simulink model "Lab1_Exercise2_BD"  (R2023b)
settings: Solver=VariableStepAuto  StartTime=0.0  StopTime=100  RelTol=1e-3
settings Model: Creator=julia  LastModifiedBy=julia

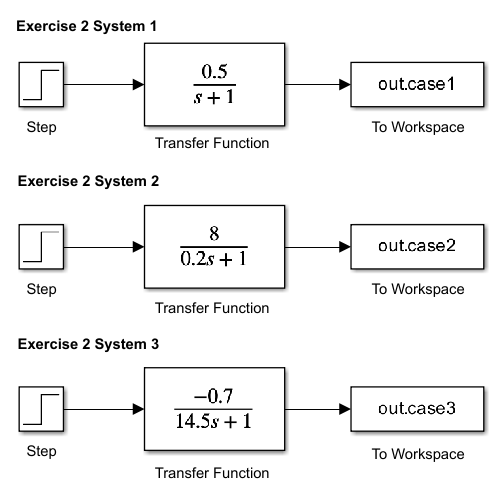
[thumbnail: Simulink's stored preview of the top-level diagram]
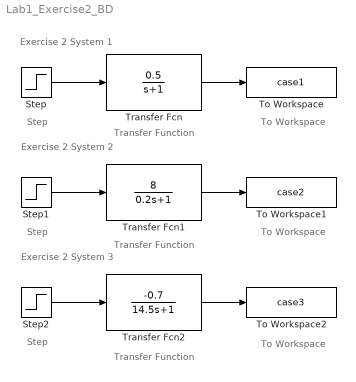
== system Lab1_Exercise2_BD ==
  note: Exercise 2 System 1
  note: Transfer Function
  note: To Workspace
  note: Step
  note: Step
  note: Step
  note: To Workspace
  note: To Workspace
  note: Transfer Function
  note: Transfer Function
  note: Exercise 2 System 2
  note: Exercise 2 System 3
  Step : Step  SampleTime=0
  Step1 : Step  SampleTime=0
  Step2 : Step  SampleTime=0
  To Workspace : ToWorkspace  VariableName=case1  SampleTime=-1
  To Workspace1 : ToWorkspace  VariableName=case2  SampleTime=-1
  To Workspace2 : ToWorkspace  VariableName=case3  SampleTime=-1
  Transfer Fcn : TransferFcn  Numerator=[0.5]  Denominator=[1 1]
  Transfer Fcn1 : TransferFcn  Numerator=[8]  Denominator=[0.2 1]
  Transfer Fcn2 : TransferFcn  Numerator=[-0.7]  Denominator=[14.5 1]
  wires:
  Step/1 -> Transfer Fcn/1
  Transfer Fcn/1 -> To Workspace/1
  Step1/1 -> Transfer Fcn1/1
  Transfer Fcn1/1 -> To Workspace1/1
  Step2/1 -> Transfer Fcn2/1
  Transfer Fcn2/1 -> To Workspace2/1
